simulink model "hbridge"  (R2024a)
settings: Solver=VariableStepAuto  StartTime=0.0  StopTime=1  RelTol=1e-3
libraries: spsMosfetLib x12, simulink x5, spsDCVoltageSourceLib x3, spsSeriesRLCBranchLib x2, spsVoltageMeasurementLib x2, sps_lib x1
settings Model: Creator=kasaa  LastModifiedBy=Aakash
settings RTWCC: GPUComputeCapability=3.5

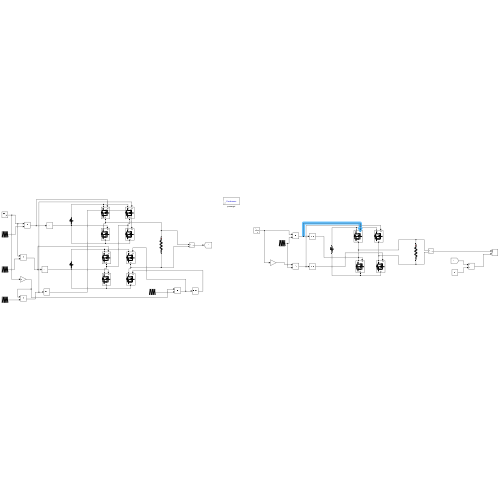
[thumbnail: Simulink's stored preview of the top-level diagram]
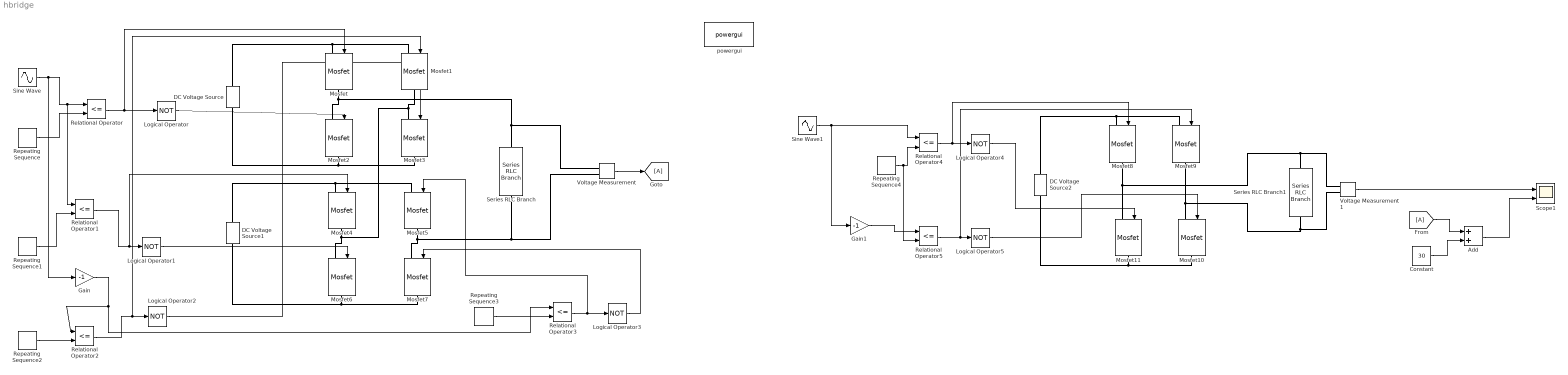
== system hbridge ==
  Add : Sum
  Constant : Constant  Value=30
  DC Voltage Source : spsDCVoltageSourceLib/DC Voltage Source  Amplitude=5  Measurements=None
  DC Voltage Source1 : spsDCVoltageSourceLib/DC Voltage Source  Amplitude=5  Measurements=None
  DC Voltage Source2 : spsDCVoltageSourceLib/DC Voltage Source  Amplitude=5  Measurements=None
  From : From
  Gain : Gain  Gain=-1
  Gain1 : Gain  Gain=-1
  Goto : Goto
  Logical Operator{,1..5} (6 alike) : Logic  Operator=NOT  AllPortsSameDT=off  OutDataTypeStr=boolean
  Mosfet{,1..11} (12 alike) : spsMosfetLib/Mosfet  Ron=0.1  Lon=0  Rd=0.01  Vfd=0  IC=0  Rs=1e5  Cs=inf  Measurements=off
  Relational Operator{,1..5} (6 alike) : RelationalOperator  Operator=<=  OutDataTypeStr=boolean  RndMeth=Simplest  InputSameDT=off
  Repeating Sequence : simulink/Sources/Repeating Sequence  rep_seq_t=[0 0.5 1]/1000  rep_seq_y=[0 1 0]
  Repeating Sequence1 : simulink/Sources/Repeating Sequence  rep_seq_t=[0 0.5 1]/1000  rep_seq_y=[1 2 1]
  Repeating Sequence2 : simulink/Sources/Repeating Sequence  rep_seq_t=[0 0.5 1]/1000  rep_seq_y=[0 1 0]
  Repeating Sequence3 : simulink/Sources/Repeating Sequence  rep_seq_t=[0 0.5 1]/1000  rep_seq_y=[1 2 1]
  Repeating Sequence4 : simulink/Sources/Repeating Sequence  rep_seq_t=[0 0.5 1]/1000  rep_seq_y=[0 1 0]
  Scope1 : Scope  NumInputPorts=2
  Series RLC Branch : spsSeriesRLCBranchLib/Series RLC Branch  LConnTagsString=__new0  RConnTagsString=__new0  BranchType=R  Resistance=100  Inductance=1e-3  SetiL0=off  InitialCurrent=0  Capacitance=1e-6  Setx0=off  InitialVoltage=0  Measurements=None
  Series RLC Branch1 : spsSeriesRLCBranchLib/Series RLC Branch  LConnTagsString=__new0  RConnTagsString=__new0  BranchType=R  Resistance=100  Inductance=1e-3  SetiL0=off  InitialCurrent=0  Capacitance=1e-6  Setx0=off  InitialVoltage=0  Measurements=None
  Sine Wave : Sin  Amplitude=3  Frequency=314.15  SampleTime=0
  Sine Wave1 : Sin  Amplitude=3  Frequency=314.15  SampleTime=0
  Voltage Measurement : spsVoltageMeasurementLib/Voltage Measurement  PhasorSimulation=off  OutputType=Complex  PSBequivalent=0
  Voltage Measurement1 : spsVoltageMeasurementLib/Voltage Measurement  PhasorSimulation=off  OutputType=Complex  PSBequivalent=0
  powergui : sps_lib/powergui  Priority=1  SimulationMode=Continuous  SampleTime=50e-6  frequency=60  Iterations=50  frequencyindice=0  Pbase=100e6  ErrMax=1e-4  UnitsV=kV  UnitsW=MW  buscounter=0  FunctionMessages=off  echomessages=off  EnableUseOfTLC=off  CurrentSourceSwitches=off  DisableSnubberDevices=off  DisableRonSwitches=off  DisableVfSwitches=off  DisplayEquations=off  AutomaticDiscreteSolvers=off  SolverType=Tustin/Backward Euler (TBE)  Interpol=off  ExternalGateDelay=off  methode=off  Ts=100  x0status=blocks  SPID=on  SwTol=0  HookPort=off  NonlinearTolerance=1e-4  nMaxIteration=100  ContinueOnMaxIteration=off  RestoreLinks=warning  ResistiveCurrentMeasurement=off  Frange=[0:2:500]  Ylog=off  Xlog=on  ShowGrid=off  save=off  variable=ZData  structure=0  ZoomFFT=off  StartTime=0.0  cycles=1  DisplayStyle=1  fundamental=60  FreqAxis=off  MaxFrequency=1000  frequencyindicesteady=1  RmsSteady=1  display=off
  wires:
  Sine Wave/1 -> Gain/1, Relational Operator1/1, Relational Operator/1
  Repeating Sequence/1 -> Relational Operator/2
  Relational Operator/1 -> Mosfet/1, Logical Operator/1
  Logical Operator/1 -> Mosfet2/1
  Repeating Sequence1/1 -> Relational Operator1/2
  Relational Operator1/1 -> Mosfet4/1, Logical Operator1/1
  Logical Operator1/1 -> Mosfet6/1
  Repeating Sequence2/1 -> Relational Operator2/2
  Gain/1 -> Relational Operator3/1, Relational Operator2/1
  Relational Operator2/1 -> Mosfet1/1, Logical Operator2/1
  Logical Operator2/1 -> Mosfet3/1
  Repeating Sequence3/1 -> Relational Operator3/2
  Relational Operator3/1 -> Mosfet5/1, Logical Operator3/1
  Logical Operator3/1 -> Mosfet7/1
  Voltage Measurement1/1 -> Scope1/1
  Sine Wave1/1 -> Relational Operator4/1, Gain1/1
  Repeating Sequence4/1 -> Relational Operator5/2, Relational Operator4/2
  Relational Operator4/1 -> Mosfet8/1, Logical Operator4/1
  Logical Operator4/1 -> Mosfet11/1
  Gain1/1 -> Relational Operator5/1
  Relational Operator5/1 -> Mosfet9/1, Logical Operator5/1
  Logical Operator5/1 -> Mosfet10/1
  Voltage Measurement/1 -> Goto/1
  From/1 -> Add/1
  Constant/1 -> Add/2
  Add/1 -> Scope1/2
  connections:
  Mosfet2/LConn1 -- Voltage Measurement/LConn1 -- Series RLC Branch/LConn1 -- Mosfet/RConn1
  Mosfet/LConn1 -- DC Voltage Source/RConn1 -- Mosfet1/LConn1
  Mosfet2/RConn1 -- DC Voltage Source/LConn1 -- Mosfet3/RConn1
  Mosfet4/LConn1 -- DC Voltage Source1/RConn1 -- Mosfet5/LConn1
  Mosfet3/LConn1 -- Mosfet6/LConn1 -- Mosfet4/RConn1 -- Mosfet1/RConn1
  Mosfet7/LConn1 -- Voltage Measurement/LConn2 -- Series RLC Branch/RConn1 -- Mosfet5/RConn1
  Mosfet6/RConn1 -- DC Voltage Source1/LConn1 -- Mosfet7/RConn1
  Mosfet11/LConn1 -- Voltage Measurement1/LConn1 -- Series RLC Branch1/LConn1 -- Mosfet8/RConn1
  Mosfet10/LConn1 -- Voltage Measurement1/LConn2 -- Series RLC Branch1/RConn1 -- Mosfet9/RConn1
  Mosfet11/RConn1 -- Mosfet10/RConn1 -- DC Voltage Source2/LConn1
  Mosfet8/LConn1 -- Mosfet9/LConn1 -- DC Voltage Source2/RConn1
